simulink model "SinglePulse_2delays_1us"  (R2014a)
settings: Solver=FixedStepDiscrete  StartTime=0.0  StopTime=0.0  FixedStep=1  RelTol=1e-3
values from neighbouring files (symbols this model uses):
  inputPulse = inputSequence ( 76*10^6, 1, 0, 0, 300*10^-9)    [generateBus.m]    (also in plotSimulinkOutput_grid.m = inputSequence(76.92307692*10^6, 1, 0,1.5*10^-6); pulseModel.m = [75.76*10^6, 10, 0, 0, 1])
libraries: opticalComponentLibrary x23
settings Model: Creator=Alexander  LastModifiedBy=Alexander

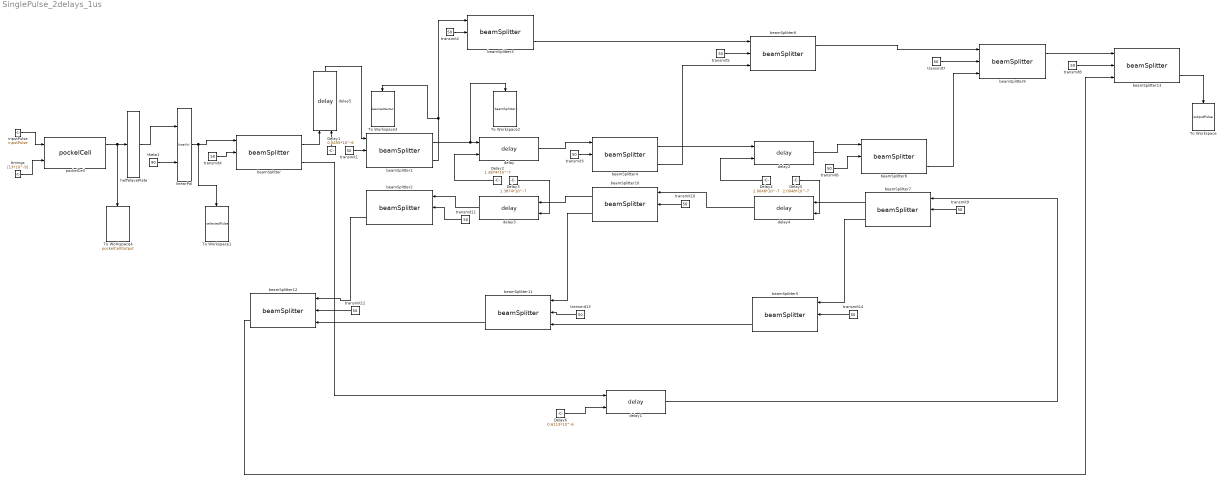
== system SinglePulse_2delays_1us ==
  Delay1 : Constant  Value=0.0495*10^-6
  Delay2 : Constant  Value=1.3874*10^-7
  Delay3 : Constant  Value=1.3874*10^-7
  Delay4 : Constant  Value=2.0048*10^-7
  Delay5 : Constant  Value=2.0048*10^-7
  Delay6 : Constant  Value=0.6113*10^-6
  To Workspace : ToWorkspace  VariableName=outputPulse  SampleTime=-1
  To Workspace1 : ToWorkspace  VariableName=selectedPulse  SampleTime=-1
  To Workspace2 : ToWorkspace  VariableName=beamSplitter1  SampleTime=-1
  To Workspace3 : ToWorkspace  VariableName=beamSplitterOut  SampleTime=-1
  To Workspace4 : ToWorkspace  VariableName=pockelCellOutput  SampleTime=-1
  beamSplitter{,1..13} (14 alike) : opticalComponentLibrary/beamSplitter
  delay{,1..5} (6 alike) : opticalComponentLibrary/delay
  halfWavePlate : opticalComponentLibrary/halfWavePlate
  inputPulse : Constant  Value=inputPulse
  linearPol : opticalComponentLibrary/linearPol
  pockelCell : opticalComponentLibrary/pockelCell
  theta1 : Constant  Value=90
  timings : Constant  Value=[13*10^-9]  SampleTime=inf
  transmit{1..14} (14 alike) : Constant  Value=50
  wires:
  pockelCell/1 -> To Workspace4/1, halfWavePlate/1
  halfWavePlate/1 -> linearPol/1
  linearPol/1 -> To Workspace1/1, beamSplitter/1
  beamSplitter/2 -> delay1/1
  delay/1 -> beamSplitter4/1
  beamSplitter1/1 -> To Workspace2/1, delay/1
  beamSplitter4/1 -> delay2/1
  beamSplitter4/2 -> beamSplitter6/3
  beamSplitter3/2 -> beamSplitter6/1
  delay4/1 -> beamSplitter10/1
  beamSplitter10/1 -> delay3/1
  delay3/1 -> beamSplitter2/1
  delay2/1 -> beamSplitter8/1
  beamSplitter6/1 -> beamSplitter9/1
  beamSplitter8/2 -> beamSplitter9/3
  delay1/1 -> beamSplitter7/1
  beamSplitter7/1 -> delay4/1
  beamSplitter7/2 -> beamSplitter5/1
  beamSplitter10/2 -> beamSplitter11/1
  beamSplitter5/2 -> beamSplitter11/3
  beamSplitter11/2 -> beamSplitter12/3
  beamSplitter2/2 -> beamSplitter12/1
  beamSplitter12/2 -> beamSplitter13/3
  beamSplitter9/1 -> beamSplitter13/1
  beamSplitter1/2 -> beamSplitter3/1, To Workspace3/1
  inputPulse/1 -> pockelCell/1
  timings/1 -> pockelCell/2
  theta1/1 -> linearPol/2
  Delay3/1 -> delay3/2
  Delay2/1 -> delay/2
  Delay4/1 -> delay2/2
  Delay5/1 -> delay4/2
  Delay6/1 -> delay1/2
  transmit4/1 -> beamSplitter/2
  transmit1/1 -> beamSplitter1/2
  transmit2/1 -> beamSplitter3/2
  transmit3/1 -> beamSplitter4/2
  transmit5/1 -> beamSplitter6/2
  transmit6/1 -> beamSplitter8/2
  transmit7/1 -> beamSplitter9/2
  transmit8/1 -> beamSplitter13/2
  transmit9/1 -> beamSplitter7/2
  transmit10/1 -> beamSplitter10/2
  transmit11/1 -> beamSplitter2/2
  transmit12/1 -> beamSplitter12/2
  transmit13/1 -> beamSplitter11/2
  transmit14/1 -> beamSplitter5/2
  beamSplitter13/2 -> To Workspace/1
  beamSplitter/1 -> delay5/1
  delay5/1 -> beamSplitter1/1
  Delay1/1 -> delay5/2
